simulink model "MCC"  (R2022b)
settings: Solver=ode15s  StartTime=0.0  StopTime=2  RelTol=1e-3
PreLoadFcn:
  | J = 3.2284*10e-6;
  | b = 3.5077*10e-6;
  | C = 0;
  | Cr = 0;
  | K = 0.0274;
  | Ke = 0.0274;
  | Kt = 0.0274;
  | R = 4;
  | L = 2.75*10e-6;
  | U = 0;
  | E = 0;
  | theta = 0;
settings Model: Creator=Youssef ABLALI  LastModifiedBy=Youssef ABLALI

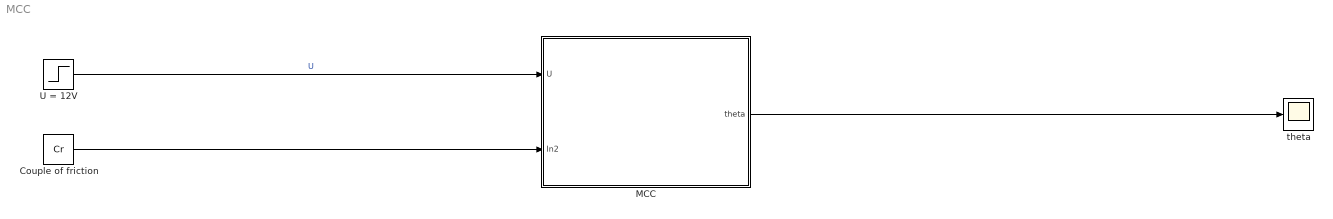
== system MCC ==
  Couple of friction : Constant  Value=Cr
  MCC : Subsystem
  U = 12V : Step  Time=0  After=12  SampleTime=0
  theta : Scope
  wires:
  U = 12V/1 -> MCC/1(U)  "U"
  Couple of friction/1 -> MCC/2(In2)
  MCC/1(theta) -> theta/1

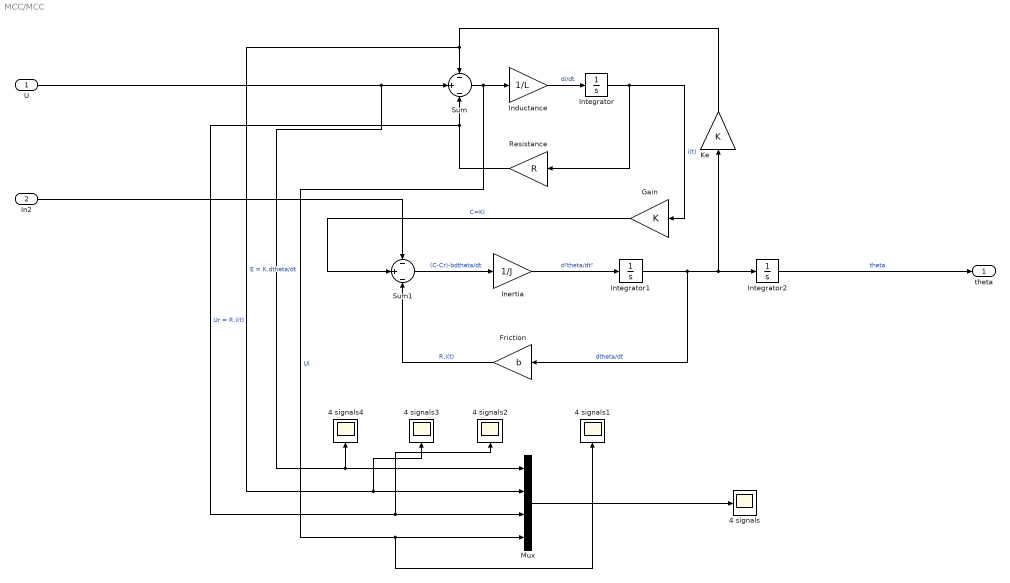
== system MCC/MCC ==
  U : Inport
  In2 : Inport  Port=2
  4 signals{,1..4} (5 alike) : Scope
  Friction : Gain  Gain=b
  Gain : Gain  Gain=K
  Inductance : Gain  Gain=1/L
  Inertia : Gain  Gain=1/J
  Integrator : Integrator
  Integrator1 : Integrator
  Integrator2 : Integrator
  Ke : Gain  Gain=K
  Mux : Mux
  Resistance : Gain  Gain=R
  Sum : Sum  Inputs=-|+|-
  Sum1 : Sum  Inputs=-|+|-
  theta : Outport
  wires:
  In2/1 -> Sum1/1
  Ke/1 -> Mux/2, 4 signals3/1, Sum/1  "E = K.dtheta/dt"
  Integrator/1 -> Gain/1, Resistance/1  "i(t)"
  Inductance/1 -> Integrator/1  "di/dt"
  Mux/1 -> 4 signals/1
  U/1 -> Sum/2, 4 signals4/1, Mux/1
  Inertia/1 -> Integrator1/1  "d²theta/dt²"
  Sum1/1 -> Inertia/1  "(C-Cr)-bdtheta/dt"
  Integrator1/1 -> Ke/1, Integrator2/1, Friction/1  "dtheta/dt"
  Sum/1 -> 4 signals1/1, Mux/4, Inductance/1  "Ul"
  Resistance/1 -> 4 signals2/1, Mux/3, Sum/3  "Ur = R.i(t)"
  Gain/1 -> Sum1/2  "C=KI"
  Friction/1 -> Sum1/3  "R.i(t)"
  Integrator2/1 -> theta/1  "theta"
